simulink library "Hub_Axis_Lib"  (Simulink 7.9)
settings: Solver=ode45  StartTime=0.0  StopTime=10.0  RelTol=1e-3
undefined symbols (not defined in the file): gcbh, mech_rtmsupport, mech_support
libraries: mblibv1 x6, fl_lib x4, nesl_utility x4, Hub_Axis_Lib x1
Description:
  | Copyright 2011 MathWorks, Inc.
settings Model: Creator=smiller  LastModifiedBy=smiller

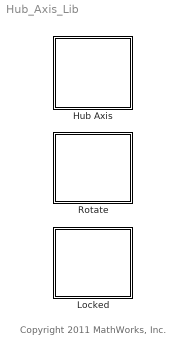
== system Hub_Axis_Lib ==
  note: Copyright 2011 MathWorks, Inc.
  Hub Axis : Subsystem  BlockChoice=Locked
      settings: TemplateBlock=self  MemberBlocks=Locked,Rotate
  Locked : Subsystem
      mask Display: image(imread('Hub_Axis_Locked_IMAGE.jpg'));
  Rotate : Subsystem
      mask Display: image(imread('Hub_Axis_Rotate_IMAGE.jpg'));

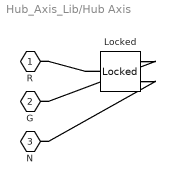
== system Hub_Axis_Lib/Hub Axis ==
  Locked : Hub_Axis_Lib/Locked  SystemSampleTime=-1
  R : PMIOPort  Port=1  Side=Left
  G : PMIOPort  Port=2  Side=Right
  N : PMIOPort  Port=3  Side=Right
  connections:
  Locked/LConn1 -- R/RConn1
  Locked/RConn1 -- G/RConn1
  Locked/RConn2 -- N/RConn1

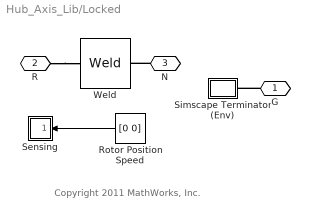
== system Hub_Axis_Lib/Locked ==
  note: Copyright 2011 MathWorks, Inc.
  Rotor Position Speed : Constant  Value=[0 0]
  Sensing : Subsystem
      mask Display: disp('S');
  Simscape Terminator (Env) : Subsystem
      mask Display:
      | plot([0 0.9],[0.5 0.5]);
      | plot([0.5 0.9],[0.3 0.3]);
      | plot([0.5 0.9],[0.7 0.7]);
      | plot([0.9 0.9],[0.7 0.3]);
  Weld : mblibv1/Joints/Weld  LConnTagsString=__newl0  RConnTagsString=__newr0  UpdateFromCAD=off  NumSAPorts=0  CutJoint=off  MarkAsCut=off  Primitives=weld  PrimitiveProps=W$WORLD$[0 0 0]$weld  DialogClass=JointBlock  WAxis=[0 0 0]
  G : PMIOPort  Port=1  Side=Right
  R : PMIOPort  Port=2  Side=Left
  N : PMIOPort  Port=3  Side=Right
  wires:
  Rotor Position Speed/1 -> Sensing/1(In1)
  connections:
  G/RConn1 -- Simscape Terminator (Env)/LConn1
  N/RConn1 -- Weld/RConn1
  R/RConn1 -- Weld/LConn1

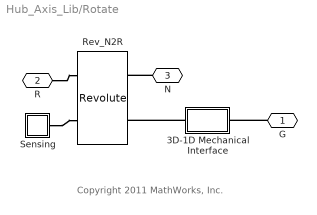
== system Hub_Axis_Lib/Rotate ==
  note: Copyright 2011 MathWorks, Inc.
  3D-1D Mechanical Interface : Subsystem
  Rev_N2R : mblibv1/Joints/Revolute  LConnTagsString=__newl0|SA1  RConnTagsString=__newr0|SA1  UpdateFromCAD=off  NumSAPorts=2  CutJoint=off  MarkAsCut=off  Primitives=prismatic  PrimitiveProps=R1$Base$[-1 0 0]$revolute  DialogClass=JointBlock  R1Axis=[-1 0 0]
  Sensing : Subsystem
  G : PMIOPort  Port=1  Side=Right
  R : PMIOPort  Port=2  Side=Left
  N : PMIOPort  Port=3  Side=Right
  connections:
  R/RConn1 -- Rev_N2R/LConn1
  N/RConn1 -- Rev_N2R/RConn1
  3D-1D Mechanical Interface/RConn1 -- Rev_N2R/RConn2
  Sensing/LConn1 -- Rev_N2R/LConn2
  G/RConn1 -- 3D-1D Mechanical Interface/LConn1

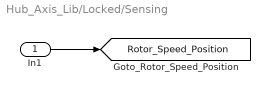
== system Hub_Axis_Lib/Locked/Sensing ==
  In1 : Inport
  tag scope: Rotor_Speed_Position=global
  wires:
  In1/1 -> [Rotor_Speed_Position]

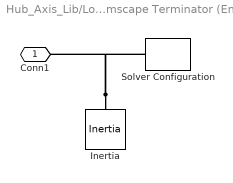
== system Hub_Axis_Lib/Locked/Simscape Terminator (Env) ==
  Inertia : fl_lib/Mechanical/Rotational Elements/Inertia  inertia=1.5e-3 kg*m^2  initial_velocity=0 rad/s  t_Log=off  LocalVarNames=|t  LocalVarDescs=|t  LocalVarLogging=0
  Solver Configuration : nesl_utility/Solver Configuration  PhysicalDomain=network_engine_domain  LeftPortType=input  RightPortType=generic  SubClassName=solver  UseCustomDae=off  DoDC=off  ResidualTolerance=1e-9  UseLocalSolver=off  LocalSolverChoice=NE_BACKWARD_EULER_ADVANCER  LocalSolverSampleTime=.001  DoFixedCost=off  MaxNonlinIter=3  MaxModeIter=2  LinearAlgebra=Sparse  Accelerate=off  Profile=off  UseLocalSampling=off  DelaysMemoryBudget=1024
  Conn1 : PMIOPort  Port=1  Side=Left
  connections:
  Inertia/LConn1 -- Conn1/RConn1 -- Solver Configuration/RConn1

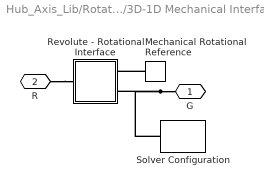
== system Hub_Axis_Lib/Rotate/3D-1D Mechanical Interface ==
  Mechanical Rotational Reference : fl_lib/Mechanical/Rotational Elements/Mechanical Rotational Reference  t_Log=off  LocalVarNames=|t  LocalVarDescs=|t  LocalVarLogging=0
  Revolute - Rotational Interface : Subsystem  DialogController=MECH.DynMechDlgSource  LoadFcn=mech_rtmsupport('LoadFcn',gcbh);mech_support('LoadFcn',gcbh);  StartFcn=mech_support('StartFcn',gcbh);  StopFcn=mech_support('StopFcn',gcbh);  mask(Revolute - Rotational Interface){UpdateFromCAD=off, PMImportedID=, ClassName=RevoluteRotationalInterface, DialogClass=RevoluteRotationalInterface, Primitive=R1}
      mask prompts: UpdateFromCAD "UPDATE_FROM_CAD"; PMImportedID "PMIMPORTED_ID"; Primitive "Connected to primitive :"
      mask help:
      | Connects a revolute primitive in the Joint attached at port R to any two mechanical rotational nodes in a Simscape network. Exchanges rotational kinetic energy between a machine and a network without loss. The base (B) and follower (F) ports correspond to the same ports on the Joint. Connect to Joint block to see Connected to primitive list.
      |
      | To ensure model validity, do not place inertia elements in interfaced Simscape circuit.
      mask init:
      | mech_preinitmask ();
      | mech_support('MaskInit',gcbh)
      settings: CopyFcn=mech_rtmsupport('CopyFcn',gcbh);mech_support('CopyFcn',gcbh);  DeleteFcn=mech_rtmsupport('DeleteFcn',gcbh);mech_support('DeleteFcn',gcbh);  UndoDeleteFcn=mech_support('UndoDeleteFcn',gcbh);  ModelCloseFcn=mech_rtmsupport('ModelCloseFcn',gcbh);mech_support('ModelCloseFcn',gcbh);  PreSaveFcn=mech_rtmsupport('PreSaveFcn',gcbh);  PostSaveFcn=mech_rtmsupport('PostSaveFcn',gcbh);  NameChangeFcn=mech_support('NameChangeFcn',gcbh);  PreCopyFcn=mech_rtmsupport('PreCopyFcn',gcbh);  CloseFcn=mech_support('CloseFcn',gcbh);  PreDeleteFcn=mech_rtmsupport('PreDeleteFcn',gcbh);
      mask Help: web(mech_help('revoluterotationalinterface'))
      mask Display: image(mech_getIcon('revolute_interface.bmp', 'Mechanical'),'center','on');color('magenta');port_label('lconn',1,'B');port_label('lconn',2,'F');color('black');port_label('rconn',1,'R');
  Solver Configuration : nesl_utility/Solver Configuration  PhysicalDomain=network_engine_domain  LeftPortType=input  RightPortType=generic  SubClassName=solver  UseCustomDae=off  DoDC=off  ResidualTolerance=WT_Params.Geartrain.Solver_Consistency_Tolerance  UseLocalSolver=off  LocalSolverChoice=NE_BACKWARD_EULER_ADVANCER  LocalSolverSampleTime=.001  DoFixedCost=off  MaxNonlinIter=3  MaxModeIter=2  LinearAlgebra=Sparse  Accelerate=off  Profile=off  UseLocalSampling=off  DelaysMemoryBudget=1024
  G : PMIOPort  Port=1  Side=Left
  R : PMIOPort  Port=2  Side=Right
  connections:
  G/RConn1 -- Revolute - Rotational Interface/LConn2 -- Solver Configuration/RConn1
  Mechanical Rotational Reference/LConn1 -- Revolute - Rotational Interface/LConn1
  R/RConn1 -- Revolute - Rotational Interface/RConn1

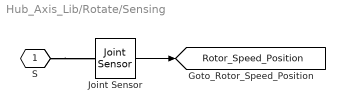
== system Hub_Axis_Lib/Rotate/Sensing ==
  Joint Sensor : mblibv1/Sensors &  Actuators/Joint Sensor  UpdateFromCAD=off  PhysicalDomain=Mechanical  PortType=blob  Muxed=on  Pose=off  Angle=on  AngleUnits=rad  ArcVelocity=on  ArcVelocityUnits=rad/s  ArcAcceleration=off  ArcAccelerationUnits=deg/s^2  CoordPosition=on  CoordPositionUnits=m  Velocity=off  VelocityUnits=m/s  Acceleration=off  AccelerationUnits=m/s^2  Quaternion=on  QuaternionDT=off  QuaternionDDT=off  QuaternionUnits=off  OutputVector=[1]  ActiveIO=off  Width=2  DialogClass=MechanicalSensorBlock  Primitive=R1  Force=off  ForceUnits=N  Torque=off  TorqueUnits=N*m  ReferenceFrame=Absolute (World)  ReactionSensedSide=Base  ReactionReferenceFrame=Absolute (World)  ReactionForce=off  ReactionForceUnits=N  ReactionMoment=off  ReactionMomentUnits=N*m
  S : PMIOPort  Tag=PMCPort  Port=1  Side=Left
  tag scope: Rotor_Speed_Position=global
  wires:
  Joint Sensor/1 -> [Rotor_Speed_Position]
  connections:
  S/RConn1 -- Joint Sensor/LConn1

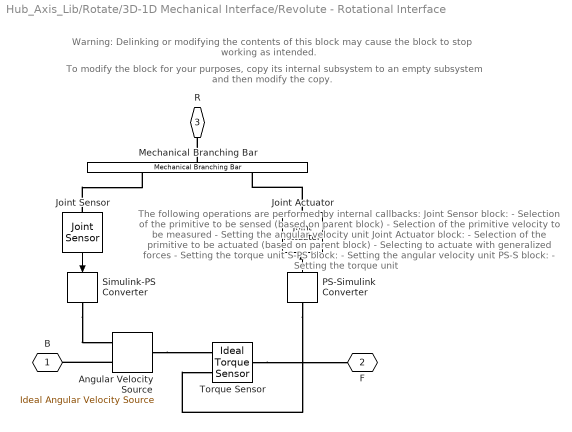
== system Hub_Axis_Lib/Rotate/3D-1D Mechanical Interface/Revolute - Rotational Interface ==
  note: Warning: Delinking or modifying the contents of
      | this block may cause the block to stop working as intended.
  note: To modify the block for your purposes, copy its internal subsystem
      | to an empty subsystem and then modify the copy.
  note: The following operations are performed by internal callbacks:
      |
      | Joint Sensor block:
      |    - Selection of the primitive to be sensed (based on parent block)
      |    - Selection of the primitive velocity to be measured
      |    - Setting the angular velocity unit
      |
      | Joint Actuator block:
      |    - Selection of the primitive to be actuated (based on parent block)
      |    - Selecting to actuate with generalized forces
      |    - Setting the torque unit
      |
      | S-PS block:
      |    - Setting the angular velocity unit
      |
      | PS-S block:
      |    - Setting the torque unit
  Angular Velocity Source : fl_lib/Mechanical/Mechanical Sources/Ideal Angular Velocity Source  w_Log=off  t_Log=off  LocalVarNames=|torque|rel_velocity|power  LocalVarDescs=|Torque (N*m)|Relative velocity (rad/s)|Power generated by the sourcec(W)  LocalVarLogging=[0 0 0]
  Joint Actuator : mblibv1/Sensors &  Actuators/Joint Actuator  UpdateFromCAD=off  PhysicalDomain=Mechanical  PortType=blob  ActuationStyle=Force  AngleUnits=deg  ArcVelocityUnits=deg/s  ArcAccelerationUnits=deg/s^2  CoordPositionUnits=m  VelocityUnits=m/s  AccelerationUnits=m/s^2  ForceUnits=N  TorqueUnits=N*m  ActiveIO=off  Width=1  DialogClass=MechanicalActuatorBlock  Primitive=R1  ReferenceFrame=Absolute (World)
  Joint Sensor : mblibv1/Sensors &  Actuators/Joint Sensor  UpdateFromCAD=off  PhysicalDomain=Mechanical  PortType=blob  Muxed=on  Pose=off  Angle=off  AngleUnits=deg  ArcVelocity=on  ArcVelocityUnits=rad/s  ArcAcceleration=off  ArcAccelerationUnits=deg/s^2  CoordPosition=off  CoordPositionUnits=m  Velocity=off  VelocityUnits=m/s  Acceleration=off  AccelerationUnits=m/s^2  Quaternion=off  QuaternionDT=off  QuaternionDDT=off  QuaternionUnits=off  OutputVector=[1]  ActiveIO=off  Width=1  DialogClass=MechanicalSensorBlock  Primitive=R1  Force=off  ForceUnits=N  Torque=off  TorqueUnits=N*m  ReferenceFrame=Absolute (World)  ReactionSensedSide=Base  ReactionReferenceFrame=Absolute (World)  ReactionForce=off  ReactionForceUnits=N  ReactionMoment=off  ReactionMomentUnits=N*m
  Mechanical Branching Bar : mblibv1/Utilities/Mechanical Branching Bar  LConnTagsString=_newl0  RConnTagsString=SA0|SA1  UpdateFromCAD=off  DialogClass=MechanicalBranchingBarBlock  NumSAPorts=2
  PS-Simulink Converter : nesl_utility/PS-Simulink Converter  PhysicalDomain=network_engine_domain  LeftPortType=input  RightPortType=output  SubClassName=ps_output  Unit=N*m  AffineConversion=off
  Simulink-PS Converter : nesl_utility/Simulink-PS Converter  PhysicalDomain=network_engine_domain  LeftPortType=input  RightPortType=output  SubClassName=ps_input  Unit=rad/s  AffineConversion=off  InputFilterTimeConstant=.001  UdotUserProvided=1  SimscapeFilterOrder=1  InputFiltering=on
  Torque Sensor : fl_lib/Mechanical/Mechanical Sensors/Ideal Torque Sensor  w_Log=off  t_Log=off  LocalVarNames=|w|t  LocalVarDescs=|w|t  LocalVarLogging=[]
  B : PMIOPort  Port=1  Side=Left
  F : PMIOPort  Port=2  Side=Left
  R : PMIOPort  Port=3  Side=Right
  wires:
  PS-Simulink Converter/1 -> Joint Actuator/1
  Joint Sensor/1 -> Simulink-PS Converter/1
  connections:
  Joint Actuator/RConn1 -- Mechanical Branching Bar/RConn2
  Joint Sensor/LConn1 -- Mechanical Branching Bar/RConn1
  Mechanical Branching Bar/LConn1 -- R/RConn1
  Torque Sensor/LConn1 -- F/RConn1
  Simulink-PS Converter/RConn1 -- Angular Velocity Source/RConn1
  Angular Velocity Source/RConn2 -- B/RConn1
  Angular Velocity Source/LConn1 -- Torque Sensor/RConn1
  PS-Simulink Converter/LConn1 -- Torque Sensor/RConn2
